simulink model "Heater"  (R2016b)
settings: Solver=VariableStepAuto  StartTime=0.0  StopTime=300  FixedStep=1  RelTol=1e-3
libraries: simulink x1
settings Model: Creator=JEDDELAN  LastModifiedBy=JEDDELAN
settings OptimizationCC: DefaultParameterBehavior=Inlined
settings DebuggingCC: ParameterTunabilityLossMsg=error
settings RTWCC: SystemTargetFile=ert.tlc  TemplateMakefile=ert_default_tmf  Description=Embedded Coder  GenerateReport=on  IncludeHyperlinkInReport=on  LaunchReport=on  GenerateTraceInfo=on  GenerateTraceReport=on  GenerateTraceReportSl=on  GenerateTraceReportSf=on  GenerateTraceReportEml=on
settings CodeAppCC: ForceParamTrailComments=on  IgnoreCustomStorageClasses=off  OperatorAnnotations=on  SimulinkDataObjDesc=on  SFDataObjDesc=on  MATLABFcnDesc=on  InsertBlockDesc=on  MATLABSourceComments=on
settings ERTTargetCC: TargetLangStandard=C99 (ISO)  GenerateSampleERTMain=on  SupportContinuousTime=on  InlinedParameterPlacement=NonHierarchical  ERTCustomFileTemplate=example_file_process.tlc

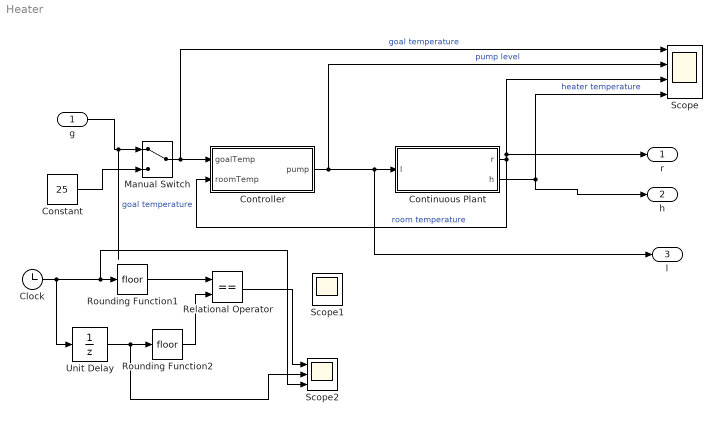
== system Heater ==
  g : Inport
  Clock : Clock
  Constant : Constant  Value=25
  Continuous Plant : Subsystem
  Controller : Subsystem
  Manual Switch : ManualSwitch
  Relational Operator : RelationalOperator  Operator===  OutDataTypeStr=boolean  RndMeth=Simplest
  Rounding Function1 : Rounding
  Rounding Function2 : Rounding
  Scope : Scope  NumInputPorts=4
  Scope1 : Scope
  Scope2 : Scope  NumInputPorts=3
  Unit Delay : UnitDelay  SampleTime=-1
  r : Outport
  h : Outport  Port=2
  l : Outport  Port=3
  wires:
  Controller/1(pump) -> Scope/2, l/1, Continuous Plant/1(l)  "pump level"
  Continuous Plant/1(r) -> Scope/3, r/1, Controller/2(roomTemp)  "room temperature"
  Continuous Plant/2(h) -> Scope/4, h/1  "heater temperature"
  Constant/1 -> Manual Switch/2
  Manual Switch/1 -> Scope/1, Controller/1(goalTemp)  "goal temperature"
  g/1 -> Manual Switch/1  "goal temperature"
  Clock/1 -> Unit Delay/1, Scope2/3, Rounding Function1/1
  Relational Operator/1 -> Scope2/1
  Rounding Function1/1 -> Relational Operator/1
  Unit Delay/1 -> Scope2/2, Rounding Function2/1
  Rounding Function2/1 -> Relational Operator/2

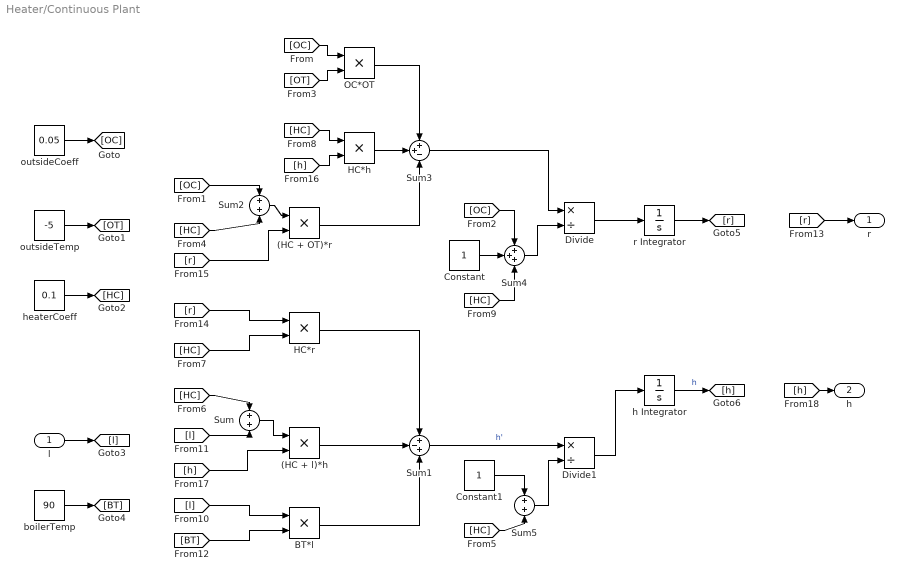
== system Heater/Continuous Plant ==
  l : Inport
  (HC + OT)*r : Product
  (HC + l)*h : Product
  BT*l : Product
  Constant : Constant
  Constant1 : Constant
  Divide : Product  Inputs=*/
  Divide1 : Product  Inputs=*/
  HC*h : Product
  HC*r : Product
  OC*OT : Product
  Sum : Sum
  Sum1 : Sum  Inputs=+-+
  Sum2 : Sum
  Sum3 : Sum  Inputs=++-
  Sum4 : Sum  Inputs=+++
  Sum5 : Sum
  boilerTemp : Constant  Value=90
  h Integrator : Integrator  InitialCondition=20
  heaterCoeff : Constant  Value=0.1
  outsideCoeff : Constant  Value=0.05
  outsideTemp : Constant  Value=-5
  r Integrator : Integrator  InitialCondition=-5
  r : Outport
  h : Outport  Port=2
  wires:
  Sum/1 -> (HC + l)*h/1
  HC*r/1 -> Sum1/1
  (HC + l)*h/1 -> Sum1/2
  BT*l/1 -> Sum1/3
  Sum2/1 -> (HC + OT)*r/1
  HC*h/1 -> Sum3/2
  OC*OT/1 -> Sum3/1
  (HC + OT)*r/1 -> Sum3/3
  Sum3/1 -> Divide/1
  Divide/1 -> r Integrator/1
  Constant/1 -> Sum4/2
  Sum4/1 -> Divide/2
  Sum1/1 -> Divide1/1  "h'"
  Sum5/1 -> Divide1/2
  Divide1/1 -> h Integrator/1
  outsideCoeff/1 -> [OC]
  [OC] -> OC*OT/1
  outsideTemp/1 -> [OT]
  [OC] -> Sum2/1
  [OC] -> Sum4/1
  [OT] -> OC*OT/2
  heaterCoeff/1 -> [HC]
  [HC] -> Sum2/2
  [HC] -> Sum5/2
  [HC] -> Sum/1
  [HC] -> HC*r/2
  [HC] -> HC*h/1
  [HC] -> Sum4/3
  l/1 -> [l]
  [l] -> BT*l/1
  [l] -> Sum/2
  boilerTemp/1 -> [BT]
  [BT] -> BT*l/2
  r Integrator/1 -> [r]
  [r] -> r/1
  [r] -> HC*r/1
  [r] -> (HC + OT)*r/2
  h Integrator/1 -> [h]  "h"
  [h] -> HC*h/2
  [h] -> (HC + l)*h/2
  [h] -> h/1
  Constant1/1 -> Sum5/1

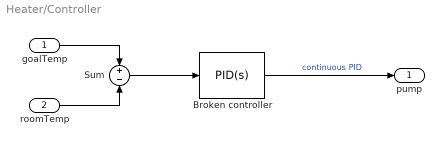
== system Heater/Controller ==
  goalTemp : Inport
  roomTemp : Inport  Port=2
  Broken controller : simulink/Continuous/PID Controller  Controller=PID  TimeDomain=Continuous-time  SampleTime=-1  IntegratorMethod=Forward Euler  FilterMethod=Forward Euler  Form=Parallel  UseFilter=off  ControllerParametersSource=internal  P=0.005  I=1.14468896e-4  D=0.005  N=100  InitialConditionSource=internal  InitialConditionForIntegrator=0  InitialConditionForFilter=0  ExternalReset=none  LimitOutput=on  UpperSaturationLimit=1  LowerSaturationLimit=0  LinearizeAsGain=on  AntiWindupMode=none  Kb=1  TrackingMode=off  Kt=1  PParamMin=[]  PParamMax=[]  IParamMin=[]  IParamMax=[]  DParamMin=[]  DParamMax=[]  NParamMin=[]  NParamMax=[]  KbParamMin=[]  KbParamMax=[]  KtParamMin=[]  KtParamMax=[]  POutMin=[]  POutMax=[]  IOutMin=[]  IOutMax=[]  DOutMin=[]  DOutMax=[]  NOutMin=[]  NOutMax=[]  KbOutMin=[]  KbOutMax=[]  KtOutMin=[]  KtOutMax=[]  IntegratorOutMin=[]  IntegratorOutMax=[]  FilterOutMin=[]  FilterOutMax=[]  SumOutMin=[]  SumOutMax=[]  SumI1OutMin=[]  SumI1OutMax=[]  SumI2OutMin=[]  SumI2OutMax=[]  SumI3OutMin=[]  SumI3OutMax=[]  SumDOutMin=[]  SumDOutMax=[]  SaturationOutMin=[]  SaturationOutMax=[]  IntegratorContinuousStateAttributes=''  IntegratorStateMustResolveToSignalObject=off  IntegratorRTWStateStorageClass=Auto  FilterContinuousStateAttributes=''  FilterStateMustResolveToSignalObject=off  FilterRTWStateStorageClass=Auto  DifferentiatorICPrevScaledInput=0  DifferentiatorOutMin=[]  DifferentiatorOutMax=[]
  Sum : Sum  Inputs=+-
  pump : Outport
  wires:
  roomTemp/1 -> Sum/2
  goalTemp/1 -> Sum/1
  Sum/1 -> Broken controller/1
  Broken controller/1 -> pump/1  "continuous PID"
